simulink model "MPC_controllers_with_disturbance"  (R2018a)
settings: Solver=VariableStepAuto  StartTime=0.0  StopTime=80  RelTol=1e-3
libraries: mpclib x2, simulink x1
settings Model: Creator=Wa'el WMJ  LastModifiedBy=Wa'el WMJ
settings DataIOCC: ReturnWorkspaceOutputs=on
settings DebuggingCC: UnconnectedInputMsg=none  UnconnectedOutputMsg=none  UnconnectedLineMsg=none
settings ModelReferenceCC: EnableRefExpFcnMdlSchedulingChecks=off
settings SFSimCC: SimUseLocalCustomCode=on
settings RTWCC: Description=Generic Real-Time Target  RTWUseLocalCustomCode=on

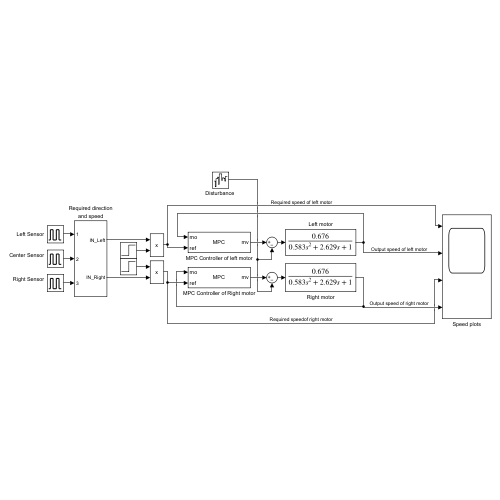
[thumbnail: Simulink's stored preview of the top-level diagram]
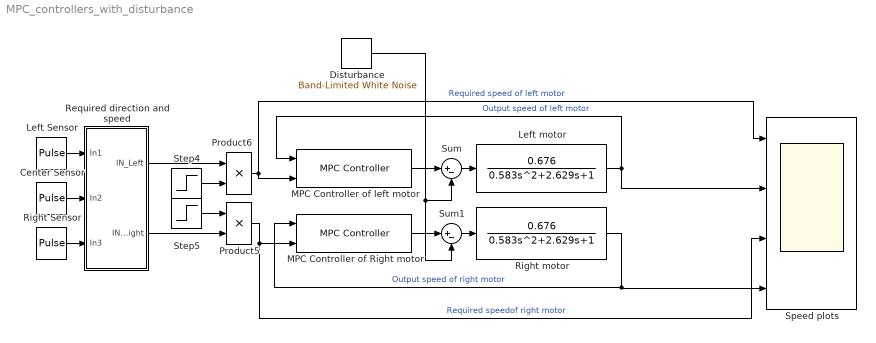
== system MPC_controllers_with_disturbance ==
  "Center Sensor " : DiscretePulseGenerator  PulseType=Time based  Period=40  PulseWidth=50  PhaseDelay=20
  "Disturbance " : simulink/Sources/Band-Limited White Noise  Cov=[20]  Ts=15  seed=[23341]
  Left Sensor : DiscretePulseGenerator  PulseType=Time based  Period=80  PulseWidth=50  PhaseDelay=40
  Left motor : TransferFcn  Numerator=[0.676]  Denominator=[0.583 2.629 1]
  MPC Controller of Right motor : mpclib/MPC Controller  SCDEnableBlockLinearizationSpecification=on  mpcobj=mpc1  is_multiple=0  enable_value=0  return_u0=off  updateMPCinCallerWorkspace=on  md_inport=off  mv_inport=off  uref_inport=off  cost_outport=off  return_sequence=off  return_qpstatus=off  return_xseq=off  return_state=off  return_ovseq=off  state_inport=off  umin_inport=off  umax_inport=off  ymin_inport=off  ymax_inport=off  cc_inport=off  ywt_inport=off  uwt_inport=off  duwt_inport=off  rhoeps_inport=off  pm_inport=off  MaximumP=10  HorizonChoice=FixedHorizon  n_ts=0.5  n_p=11  n_mv=1  n_md=0  n_ud=0  n_mo=1  n_uo=0  BlockDataType=double  SampleTimeInherited=off  switch_inport=off
  MPC Controller of left motor : mpclib/MPC Controller  SCDEnableBlockLinearizationSpecification=on  mpcobj=MPCDesigne_Left  is_multiple=0  enable_value=0  return_u0=off  updateMPCinCallerWorkspace=on  md_inport=off  mv_inport=off  uref_inport=off  cost_outport=off  return_sequence=off  return_qpstatus=off  return_xseq=off  return_state=off  return_ovseq=off  state_inport=off  umin_inport=off  umax_inport=off  ymin_inport=off  ymax_inport=off  cc_inport=off  ywt_inport=off  uwt_inport=off  duwt_inport=off  rhoeps_inport=off  pm_inport=off  MaximumP=10  HorizonChoice=FixedHorizon  n_ts=0.5  n_p=11  n_mv=1  n_md=0  n_ud=0  n_mo=1  n_uo=0  BlockDataType=double  SampleTimeInherited=off  switch_inport=off
  Product5 : Product
  Product6 : Product
  Required direction and speed : Subsystem
  "Right Sensor " : DiscretePulseGenerator  PulseType=Time based  Period=20  PulseWidth=50  PhaseDelay=10
  Right motor : TransferFcn  Numerator=[0.676]  Denominator=[0.583 2.629 1]
  Speed plots : Scope  NumInputPorts=4
  Step4 : Step  Time=0  SampleTime=0
  Step5 : Step  Time=0  SampleTime=0
  Sum : Sum  Inputs=|+-
  Sum1 : Sum  Inputs=|+-
  wires:
  Left motor/1 -> MPC Controller of left motor/1, Speed plots/2  "Output speed of left motor"
  Right motor/1 -> MPC Controller of Right motor/1, Speed plots/4  "Output speed of right motor"
  Product6/1 -> Speed plots/1, MPC Controller of left motor/2  "Required speed of left motor"
  Left Sensor/1 -> Required direction and speed/1(In1)
  Step5/1 -> Product5/1
  Required direction and speed/2(IN_Right) -> Product5/2
  "Right Sensor "/1 -> Required direction and speed/3(In3)
  Required direction and speed/1(IN_Left) -> Product6/1
  "Center Sensor "/1 -> Required direction and speed/2(In2)
  Step4/1 -> Product6/2
  Product5/1 -> Speed plots/3, MPC Controller of Right motor/2  "Required speedof right motor"
  MPC Controller of left motor/1 -> Sum/1
  Sum/1 -> Left motor/1
  "Disturbance "/1 -> Sum1/2, Sum/2
  MPC Controller of Right motor/1 -> Sum1/1
  Sum1/1 -> Right motor/1

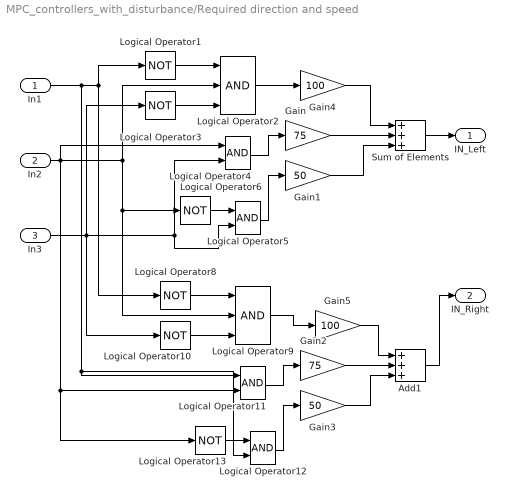
== system MPC_controllers_with_disturbance/Required direction and speed ==
  In1 : Inport
  In2 : Inport  Port=2
  In3 : Inport  Port=3
  Add1 : Sum  Inputs=+++
  Gain : Gain  Gain=75
  Gain1 : Gain  Gain=50
  Gain2 : Gain  Gain=75
  Gain3 : Gain  Gain=50
  Gain4 : Gain  Gain=100
  Gain5 : Gain  Gain=100
  Logical Operator{1,3,6,8,10,13} (6 alike) : Logic  Operator=NOT  Inputs=3  AllPortsSameDT=off  OutDataTypeStr=boolean
  Logical Operator{4..5,11..12} (4 alike) : Logic  AllPortsSameDT=off  OutDataTypeStr=boolean
  Logical Operator2 : Logic  Inputs=3  AllPortsSameDT=off  OutDataTypeStr=boolean
  Logical Operator9 : Logic  Inputs=3  AllPortsSameDT=off  OutDataTypeStr=boolean
  Sum of Elements : Sum  Inputs=+++
  IN_Left : Outport
  IN_Right : Outport  Port=2
  wires:
  Logical Operator1/1 -> Logical Operator2/1
  Logical Operator3/1 -> Logical Operator2/3
  In1/1 -> Logical Operator12/2, Logical Operator11/1, Logical Operator8/1, Logical Operator1/1
  In2/1 -> Logical Operator13/1, Logical Operator11/2, Logical Operator4/1, Logical Operator9/2, Logical Operator6/1, Logical Operator2/2
  In3/1 -> Logical Operator10/1, Logical Operator5/2, Logical Operator4/2, Logical Operator3/1
  Logical Operator6/1 -> Logical Operator5/1
  Logical Operator4/1 -> Gain/1
  Logical Operator5/1 -> Gain1/1
  Logical Operator11/1 -> Gain2/1
  Gain2/1 -> Add1/2
  Logical Operator10/1 -> Logical Operator9/3
  Logical Operator8/1 -> Logical Operator9/1
  Gain3/1 -> Add1/3
  Logical Operator12/1 -> Gain3/1
  Logical Operator13/1 -> Logical Operator12/1
  Add1/1 -> IN_Right/1
  Sum of Elements/1 -> IN_Left/1
  Gain/1 -> Sum of Elements/2
  Gain1/1 -> Sum of Elements/3
  Gain4/1 -> Sum of Elements/1
  Logical Operator2/1 -> Gain4/1
  Gain5/1 -> Add1/1
  Logical Operator9/1 -> Gain5/1
